simulink model "MOD1_CT"  (R2017a)
settings: Solver=VariableStepAuto  StartTime=0.0  StopTime=10.0  RelTol=1e-3
undefined symbols (not defined in the file): designMultirateFIR
libraries: dspmlti4 x1
settings Model: Creator=bhannigan  LastModifiedBy=bhannigan

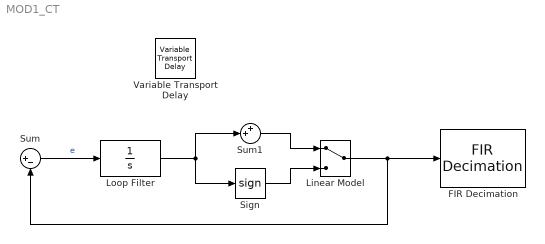
== system MOD1_CT ==
  FIR Decimation : dspmlti4/FIR Decimation  FilterSource=Auto  h=designMultirateFIR(1,2)  D=2  filtStruct=Direct form  FilterObject=FDECIM  InputProcessing=Columns as channels (frame based)  framing=Enforce single-rate processing  inputOffset=0  outputBufInitCond=0  roundingMode=Floor  overflowMode=off  firstCoeffDataTypeStr=Inherit: Same word length as input  firstCoeffMin=[]  firstCoeffMax=[]  firstCoeffLastDataTypeStr=Inherit: Same word length as input  outputDataTypeStr=Inherit: Same as accumulator  outputMin=[]  outputMax=[]  outputLastDataTypeStr=Inherit: Same as accumulator
  Linear Model : ManualSwitch
  Loop Filter : TransferFcn  Denominator=[1 0]
  Sign : Signum
  Sum : Sum  Inputs=|+-
  Sum1 : Sum  Inputs=++|
  Variable Transport Delay : VariableTransportDelay  VariableDelayType=Variable transport delay  MaximumDelay=10
  wires:
  Sum/1 -> Loop Filter/1  "e"
  Loop Filter/1 -> Sign/1, Sum1/2
  Sum1/1 -> Linear Model/1
  Sign/1 -> Linear Model/2
  Linear Model/1 -> FIR Decimation/1, Sum/2
